simulink model "Figure9"  (R2021b)
settings: Solver=VariableStepAuto  StartTime=0.0  StopTime=10.0  RelTol=1e-3
undefined symbols (not defined in the file or in its folder): get, gray, res
libraries: myLib_CustomBoolean x39, dspobslib x1
settings Model: Creator=matt  LastModifiedBy=matt

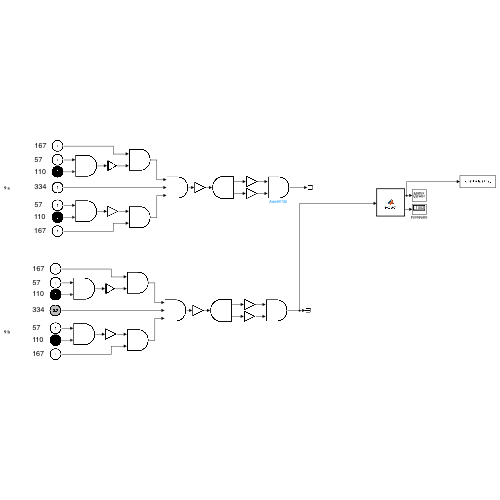
[thumbnail: Simulink's stored preview of the top-level diagram]
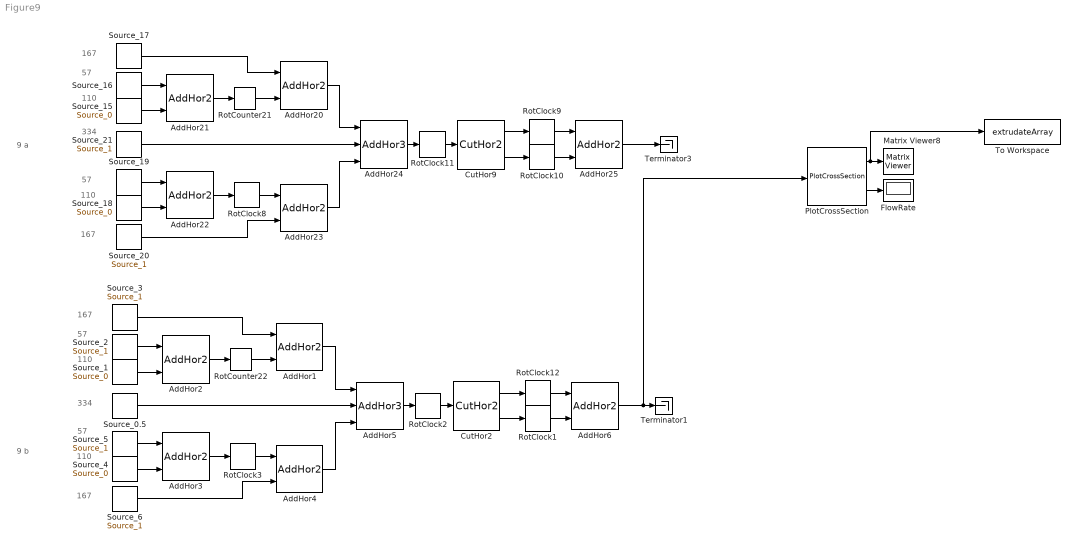
== system Figure9 ==
  note: 9 a
  note: 334
  note: 110
  note: 167
  note: 57
  note: 57
  note: 167
  note: 110
  note: 57
  note: 110
  note: 334
  note: 167
  note: 167
  note: 57
  note: 110
  note: 9 b
  AddHor{1..4,6,20..23,25} (10 alike) : myLib_CustomBoolean/AddHor2  SystemSampleTime=-1  VariantActivationTime=update diagram  Latency=0  AutoFrameSizeCalculation=off
      settings: SourceProductName=Boolean_Custom_Library
  AddHor24 : myLib_CustomBoolean/AddHor3  SystemSampleTime=-1  VariantActivationTime=update diagram  Latency=0  AutoFrameSizeCalculation=off
      settings: SourceProductName=Boolean_Custom_Library
  AddHor5 : myLib_CustomBoolean/AddHor3  SystemSampleTime=-1  VariantActivationTime=update diagram  Latency=0  AutoFrameSizeCalculation=off
      settings: SourceProductName=Boolean_Custom_Library
  CutHor2 : myLib_CustomBoolean/CutHor2  SystemSampleTime=-1  VariantActivationTime=update diagram  Latency=0  AutoFrameSizeCalculation=off
      settings: SourceProductName=Boolean_Custom_Library
  CutHor9 : myLib_CustomBoolean/CutHor2  SystemSampleTime=-1  VariantActivationTime=update diagram  Latency=0  AutoFrameSizeCalculation=off
      settings: SourceProductName=Boolean_Custom_Library
  FlowRate : Display
  Matrix Viewer8 : dspobslib/Matrix Viewer  ImageParams=off  CMapStr=gray(3)  AxisColorbar=on  AxisParams=off  AxisOrigin=Upper left corner  AxisTickMode=User-defined  XTickRange=[0 1]  YTickRange=[0 1]  XLabel=X-axis  YLabel=Y-axis  ZLabel=Z-axis  FigPos=get(0,'defaultfigureposition')  AxisZoom=off
      settings: SourceProductBaseCode=DS  YMin=0  YMax=1
  PlotCrossSection : myLib_CustomBoolean/PlotCrossSection  SystemSampleTime=-1  VariantActivationTime=update diagram  Latency=0  AutoFrameSizeCalculation=off
      settings: SourceProductName=Boolean_Custom_Library
  RotClock{1..3,8..12} (8 alike) : myLib_CustomBoolean/RotClock  SystemSampleTime=-1  VariantActivationTime=update diagram  Latency=0  AutoFrameSizeCalculation=off
      settings: SourceProductName=Boolean_Custom_Library
  RotCounter21 : myLib_CustomBoolean/RotCounter  SystemSampleTime=-1  VariantActivationTime=update diagram  Latency=0  AutoFrameSizeCalculation=off
      settings: SourceProductName=Boolean_Custom_Library
  RotCounter22 : myLib_CustomBoolean/RotCounter  SystemSampleTime=-1  VariantActivationTime=update diagram  Latency=0  AutoFrameSizeCalculation=off
      settings: SourceProductName=Boolean_Custom_Library
  Source_0.5 : myLib_CustomBoolean/Source_0.5  Value=cat(3, 0.5.*ones(res,res), 334*ones(res,res))  VectorParams1D=off  OutMin=[]  OutMax=[]  OutDataTypeStr=Inherit: Inherit from 'Constant value'  SampleTime=inf  FramePeriod=inf
      settings: SourceProductName=Boolean_Custom_Library
  Source_{1,4,15,18} (4 alike) : myLib_CustomBoolean/Source_0  Value=cat(3, 0.*ones(res,res), 110.*ones(res,res))  VectorParams1D=off  OutMin=[]  OutMax=[]  OutDataTypeStr=Inherit: Inherit from 'Constant value'  SampleTime=inf  FramePeriod=inf
      settings: SourceProductName=Boolean_Custom_Library
  Source_{2,5,16,19} (4 alike) : myLib_CustomBoolean/Source_1  Value=cat(3, 1.*ones(res,res), 57*ones(res,res))  VectorParams1D=off  OutMin=[]  OutMax=[]  OutDataTypeStr=Inherit: Inherit from 'Constant value'  SampleTime=inf  FramePeriod=inf
      settings: SourceProductName=Boolean_Custom_Library
  Source_{3,6,17,20} (4 alike) : myLib_CustomBoolean/Source_1  Value=cat(3, 1.*ones(res,res), 167*ones(res,res))  VectorParams1D=off  OutMin=[]  OutMax=[]  OutDataTypeStr=Inherit: Inherit from 'Constant value'  SampleTime=inf  FramePeriod=inf
      settings: SourceProductName=Boolean_Custom_Library
  Source_21 : myLib_CustomBoolean/Source_1  Value=cat(3, 1*ones(res,res), 334*ones(res,res))  VectorParams1D=off  OutMin=[]  OutMax=[]  OutDataTypeStr=Inherit: Inherit from 'Constant value'  SampleTime=inf  FramePeriod=inf
      settings: SourceProductName=Boolean_Custom_Library
  Terminator1 : Terminator
  Terminator3 : Terminator
  To Workspace : ToWorkspace  VariableName=extrudateArray  SampleTime=51
  wires:
  Source_5/1 -> AddHor3/1
  AddHor4/1 -> AddHor5/3
  RotClock2/1 -> CutHor2/1
  AddHor3/1 -> RotClock3/1
  RotClock12/1 -> AddHor6/1
  AddHor6/1 -> PlotCrossSection/1, Terminator1/1
  AddHor1/1 -> AddHor5/1
  Source_0.5/1 -> AddHor5/2
  AddHor5/1 -> RotClock2/1
  Source_3/1 -> AddHor1/1
  RotClock3/1 -> AddHor4/1
  CutHor2/2 -> RotClock1/1
  Source_6/1 -> AddHor4/2
  RotClock1/1 -> AddHor6/2
  AddHor2/1 -> RotCounter22/1
  Source_2/1 -> AddHor2/1
  Source_4/1 -> AddHor3/2
  RotCounter22/1 -> AddHor1/2
  CutHor2/1 -> RotClock12/1
  Source_1/1 -> AddHor2/2
  Source_17/1 -> AddHor20/1
  RotClock11/1 -> CutHor9/1
  AddHor25/1 -> Terminator3/1
  Source_16/1 -> AddHor21/1
  Source_18/1 -> AddHor22/2
  Source_20/1 -> AddHor23/2
  AddHor23/1 -> AddHor24/3
  RotClock10/1 -> AddHor25/2
  CutHor9/1 -> RotClock9/1
  AddHor20/1 -> AddHor24/1
  RotClock9/1 -> AddHor25/1
  RotCounter21/1 -> AddHor20/2
  Source_15/1 -> AddHor21/2
  AddHor22/1 -> RotClock8/1
  RotClock8/1 -> AddHor23/1
  Source_21/1 -> AddHor24/2
  CutHor9/2 -> RotClock10/1
  Source_19/1 -> AddHor22/1
  AddHor21/1 -> RotCounter21/1
  AddHor24/1 -> RotClock11/1
  PlotCrossSection/2 -> FlowRate/1
  PlotCrossSection/1 -> To Workspace/1, Matrix Viewer8/1
